simulink model "HydraulicExample"  (R2022b)
settings: Solver=VariableStepAuto  StartTime=0.0  StopTime=80  RelTol=1e-4
libraries: sh_lib x5, nesl_utility x5, fl_lib x1
settings Model: PacingRate=0.800000  Creator=user  LastModifiedBy=user

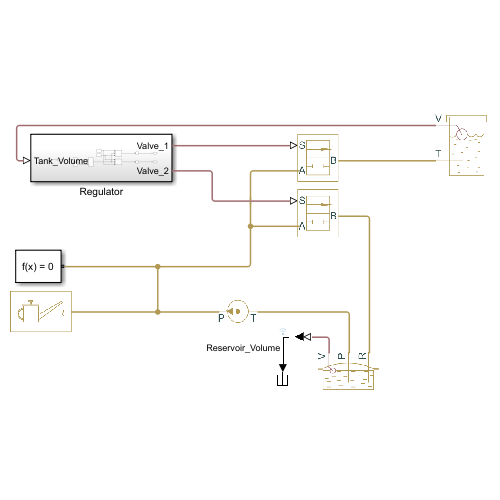
[thumbnail: Simulink's stored preview of the top-level diagram]
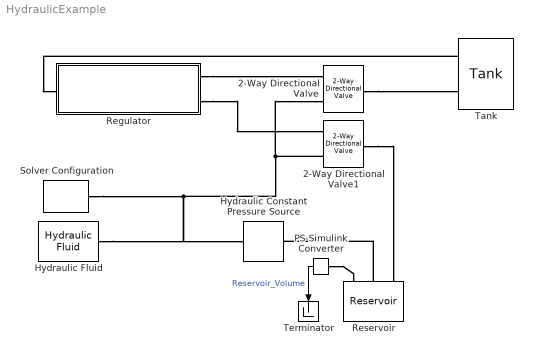
== system HydraulicExample ==
  2-Way Directional Valve : sh_lib/Valves/Directional Valves/2-Way Directional Valve  mdl_type=1  area_max=1.2e-4 m^2  opening_max=0.01 m  opening_tab=[-.002, 0, .002, .005, .015] m  area_tab=[1e-09, 2.0352e-07, 4.0736e-05, .00011438, .00034356] m^2  pressure_tab=[-10000000, -5000000, -2000000, 2000000, 5000000, 10000000] Pa  flow_rate_tab=[-1e-07, -7.0711e-08, -4.4721e-08, 4.4721e-08, 7.0711e-08, 1e-07; -2.0352e-05, -1.4391e-05, -9.1017e-06, 9.1017e-06, 1.4391e-05, 2.0352e-05; -.0040736, -.0028805, -.0018218, .0018218, .0028805, .0040736; -.011438, -.0080879, -.0051152, .0051152, .0080879, .011438; -.034356, -.024293, -.015364, .015364, .024293, .034356] m^3/s  interp_method=1  extrap_method=1  C_d=0.7  x_0=0 m  A_leak=1e-12 m^2  lam_spec=1  B_lam=0.999  Re_cr=12
      settings: InternalSimscapePortConfiguration="{\"Bottom\":[],\"Left\":[{\"id\":\"S\",\"label\":\"S\",\"type\":\"input\"},{\"id\":\"A\",\"label\":\"A\",\"type\":\"foundation.hydraulic.hydraulic\"}],\"Right\":[{\"id\":\"B\",\"label\":\"B\",\"type\":\"foundation.hydraulic.hydraulic\"}],\"Top\":[]}"
  2-Way Directional Valve1 : sh_lib/Valves/Directional Valves/2-Way Directional Valve  mdl_type=1  area_max=2.2e-4 m^2  opening_max=0.01 m  opening_tab=[-.002, 0, .002, .005, .015] m  area_tab=[1e-09, 2.0352e-07, 4.0736e-05, .00011438, .00034356] m^2  pressure_tab=[-10000000, -5000000, -2000000, 2000000, 5000000, 10000000] Pa  flow_rate_tab=[-1e-07, -7.0711e-08, -4.4721e-08, 4.4721e-08, 7.0711e-08, 1e-07; -2.0352e-05, -1.4391e-05, -9.1017e-06, 9.1017e-06, 1.4391e-05, 2.0352e-05; -.0040736, -.0028805, -.0018218, .0018218, .0028805, .0040736; -.011438, -.0080879, -.0051152, .0051152, .0080879, .011438; -.034356, -.024293, -.015364, .015364, .024293, .034356] m^3/s  interp_method=1  extrap_method=1  C_d=0.7  x_0=0 m  A_leak=1e-12 m^2  lam_spec=1  B_lam=0.999  Re_cr=12
      settings: InternalSimscapePortConfiguration="{\"Bottom\":[],\"Left\":[{\"id\":\"S\",\"label\":\"S\",\"type\":\"input\"},{\"id\":\"A\",\"label\":\"A\",\"type\":\"foundation.hydraulic.hydraulic\"}],\"Right\":[{\"id\":\"B\",\"label\":\"B\",\"type\":\"foundation.hydraulic.hydraulic\"}],\"Top\":[]}"
  Hydraulic Constant Pressure Source : fl_lib/Hydraulic/Hydraulic Sources/Hydraulic Constant Pressure Source  commanded_pressure=10e6 Pa
      settings: InternalSimscapePortConfiguration="{\"Bottom\":[],\"Left\":[{\"id\":\"P\",\"label\":\"P\",\"type\":\"foundation.hydraulic.hydraulic\"}],\"Right\":[{\"id\":\"T\",\"label\":\"T\",\"type\":\"foundation.hydraulic.hydraulic\"}],\"Top\":[]}"
  Hydraulic Fluid : sh_lib/Hydraulic Utilities/Hydraulic Fluid  SelFluid=1  SysTemp=60  TrapAir=0.005  ViscDerFactor=1  range_error=2
  PS-Simulink Converter : nesl_utility/PS-Simulink Converter  PhysicalDomain=network_engine_domain  SubClassName=ps_output  LeftPortType=input  RightPortType=output  PseudoPeriodic=off  Frequencies=[]  VectorFormat=inherit  Unit=inherit  AffineConversion=off
  Regulator : Subsystem
  Reservoir : sh_lib/Hydraulic Utilities/Reservoir  press=0 Pa  init_volume=3 m^3  ret_diam=0.02 m  loss_coeff=1
      settings: InternalSimscapePortConfiguration="{\"Bottom\":[],\"Left\":[{\"id\":\"V\",\"label\":\"V\",\"type\":\"output\"},{\"id\":\"P\",\"label\":\"P\",\"type\":\"foundation.hydraulic.hydraulic\"},{\"id\":\"R\",\"label\":\"R\",\"type\":\"foundation.hydraulic.hydraulic\"}],\"Right\":[],\"Top\":[]}"
  Solver Configuration : nesl_utility/Solver Configuration  PhysicalDomain=network_engine_domain  SubClassName=solver  LeftPortType=input  RightPortType=generic  Tones=[]  Harmonics=[]  SimulateNoise=off  Profile=off  UseLocalSampling=off  EnableSwitchedLinearOptims=on  FrequencyDomain=off  UseCCode=off  RelTol=0.001  AbsTol=0.001  MinStep=1e-09  ToWorkspace=off  RevertToSquareIcSolve=off  NumHomotopyIterations=100  PhasorMode=off  PhasorModeNumHarmonics=1  ConsistencySolver=NEWTON_XTOL_AFTER_FTOL  IndexReductionMethod=DerivativeReplacement  DoDC=off  ResidualTolerance=1e-09  ConsistencyTolSource=GLOBAL  ConsistencyAbsTol=0.001  ConsistencyRelTol=0.001  ConsistencyTolFactor=0.001  UseLocalSolver=on  LocalSolverChoice=NE_BACKWARD_EULER_ADVANCER  ResolveIndetEquations=on  FunctionEvalNumThread=1  LocalSolverSampleTime=0.001  DoFixedCost=on  MaxNonlinIter=3  MaxModeIter=2  ComputeImpulses=off  ImpulseIterations=2  LinearAlgebra=auto  LinearAlgebraNumThread=0  EquationFormulation=NE_TIME_EF  DelaysMemoryBudget=1024  AutomaticFiltering=on  FilteringTimeConstant=0.001  PartitionStorageMethod=AS_NEEDED  PartitionMemoryBudget=1024  PartitionMethod=ROBUST
  Tank : sh_lib/Low-Pressure Blocks/Tank  press=0 Pa  level_spec=1  tank_area=0.8 m^2  fluid_volume_tab=[0, .0028, .0065, .0114, .0176, .0252, .0344, .0436, .0512, .0574, .0623, .066, .0688, .0707, .072, .0727] m^3  fluid_level_tab=[0, .02, .04, .06, .08, .1, .12, .14, .16, .18, .2, .22, .24, .26, .28, .3] m  interp_method=1  extrap_method=1  pipe_diam=0.02 m  loss_coeff=1.2  g=9.80665 m/s^2  min_level=1e-3 m  fluid_level_check=0  volume_specify=on  volume_priority=High  volume=1e-5 cm^3  volume_nominal_specify=off  volume_nominal_unit=m^3  volume_nominal_value=0.3  level_specify=off  level_priority=None  level=0.025 m  level_nominal_specify=off  level_nominal_unit=m  level_nominal_value=1  pipe_diam_A=0.02 m  loss_coeff_A=1.2  height_B=0.8 m  pipe_diam_B=0.02 m  loss_coeff_B=1.2  height_C=0.8 m  pipe_diam_C=0.02 m  loss_coeff_C=1.2
      settings: InternalSimscapePortConfiguration="{\"Bottom\":[],\"Left\":[],\"Right\":[{\"id\":\"V\",\"label\":\"V\",\"type\":\"output\"},{\"id\":\"T\",\"label\":\"T\",\"type\":\"foundation.hydraulic.hydraulic\"}],\"Top\":[]}"
  Terminator : Terminator
  wires:
  PS-Simulink Converter/1 -> Terminator/1  "Reservoir_Volume"
  connections:
  2-Way Directional Valve1/LConn2 -- 2-Way Directional Valve/LConn2 -- Hydraulic Fluid/RConn1 -- Hydraulic Constant Pressure Source/LConn1 -- Solver Configuration/RConn1
  Reservoir/LConn2 -- Hydraulic Constant Pressure Source/RConn1
  2-Way Directional Valve/RConn1 -- Tank/RConn2
  2-Way Directional Valve1/RConn1 -- Reservoir/LConn3
  Tank/RConn1 -- Regulator/LConn1
  Regulator/RConn1 -- 2-Way Directional Valve/LConn1
  Regulator/RConn2 -- 2-Way Directional Valve1/LConn1
  PS-Simulink Converter/LConn1 -- Reservoir/LConn1

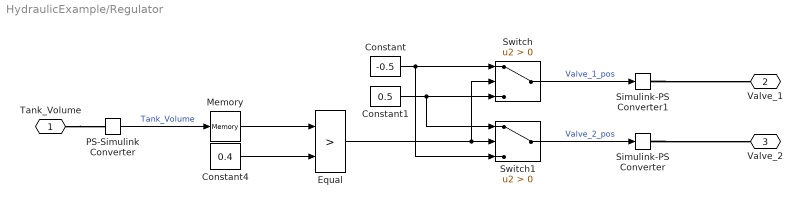
== system HydraulicExample/Regulator ==
  Constant : Constant  Value=-0.5
  Constant1 : Constant  Value=0.5
  Constant4 : Constant  Value=0.4
  Equal : RelationalOperator  Operator=>  OutDataTypeStr=boolean  RndMeth=Simplest  InputSameDT=off
  Memory : Memory
  PS-Simulink Converter : nesl_utility/PS-Simulink Converter  PhysicalDomain=network_engine_domain  SubClassName=ps_output  LeftPortType=input  RightPortType=output  PseudoPeriodic=off  Frequencies=[]  VectorFormat=inherit  Unit=inherit  AffineConversion=off
  Simulink-PS Converter : nesl_utility/Simulink-PS Converter  PhysicalDomain=network_engine_domain  SubClassName=ps_input  LeftPortType=input  RightPortType=output  PseudoPeriodic=off  Frequencies=[]  NoiseDistribution=none  NoiseParameters=[]  Unit=m  AffineConversion=off  FilteringAndDerivatives=provide  SimscapeFilterOrder=1  InputFilterTimeConstant=0.001  UdotUserProvided=0
  Simulink-PS Converter1 : nesl_utility/Simulink-PS Converter  PhysicalDomain=network_engine_domain  SubClassName=ps_input  LeftPortType=input  RightPortType=output  PseudoPeriodic=off  Frequencies=[]  NoiseDistribution=none  NoiseParameters=[]  Unit=m  AffineConversion=off  FilteringAndDerivatives=provide  SimscapeFilterOrder=1  InputFilterTimeConstant=0.001  UdotUserProvided=0
  Switch : Switch  Criteria=u2 > Threshold  SaturateOnIntegerOverflow=off  InputSameDT=off
  Switch1 : Switch  Criteria=u2 > Threshold  SaturateOnIntegerOverflow=off  InputSameDT=off
  Tank_Volume : PMIOPort  Side=Left
  Valve_1 : PMIOPort  Port=2  Side=Right
  Valve_2 : PMIOPort  Port=3  Side=Right
  wires:
  Constant1/1 -> Switch1/1, Switch/3
  Switch1/1 -> Simulink-PS Converter/1  "Valve_2_pos"
  Constant/1 -> Switch1/3, Switch/1
  Switch/1 -> Simulink-PS Converter1/1  "Valve_1_pos"
  Memory/1 -> Equal/1
  Equal/1 -> Switch1/2, Switch/2
  Constant4/1 -> Equal/2
  PS-Simulink Converter/1 -> Memory/1  "Tank_Volume"
  connections:
  Simulink-PS Converter/RConn1 -- Valve_2/RConn1
  Simulink-PS Converter1/RConn1 -- Valve_1/RConn1
  Tank_Volume/RConn1 -- PS-Simulink Converter/LConn1
